simulink model "ModeloNoLineal"  (R2024b)
settings: Solver=VariableStepAuto  StartTime=0.0  StopTime=30  RelTol=1e-3
values from neighbouring files (symbols this model uses):
  B1 = 1200    [ValoresIniciales.m]
  B2 = 500    [ValoresIniciales.m]
  Bt = 10    [ValoresIniciales.m]
  Fs = 0    [ValoresIniciales.m]
  Knl = 1.0e6    (= 1000000)    [ValoresIniciales.m]
  Ks = 16000    [ValoresIniciales.m]    (also in quarter_car_model.m = 48000)
  Kt = 160000    [ValoresIniciales.m]    (also in quarter_car_model.m = 200000)
  Mb = 300    [ValoresIniciales.m]
  Mw = 30    [ValoresIniciales.m]
settings Model: Creator=juanp  LastModifiedBy=juanp

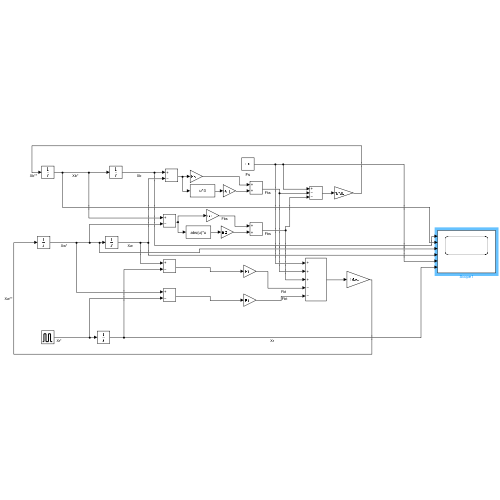
[thumbnail: Simulink's stored preview of the top-level diagram]
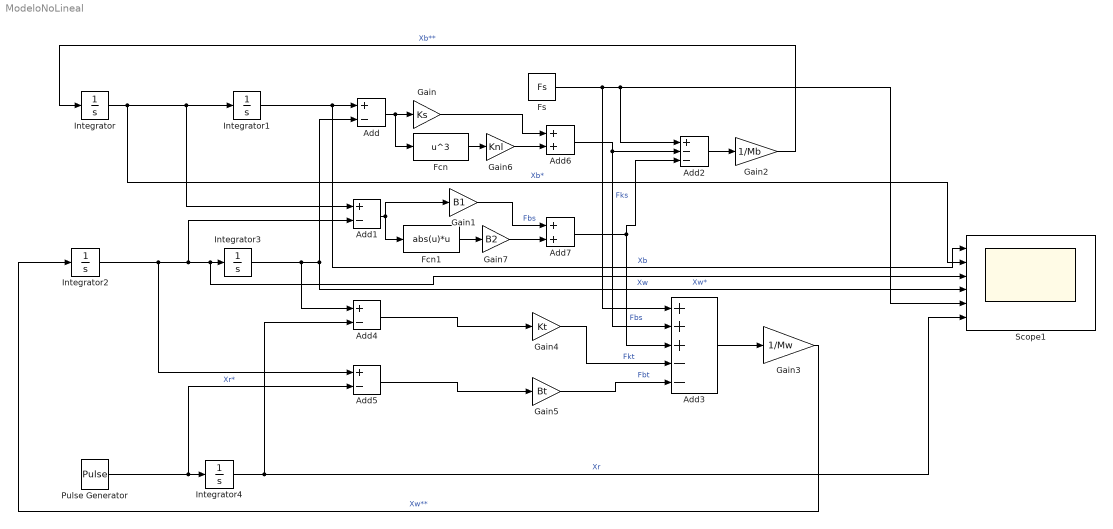
== system ModeloNoLineal ==
  Add{,1,4..5} (4 alike) : Sum  Inputs=+-
  Add2 : Sum  Inputs=+--
  Add3 : Sum  Inputs=+++--
  Add6 : Sum
  Add7 : Sum
  Fcn : Fcn  Expr=u^3
  Fcn1 : Fcn  Expr=abs(u)*u
  Fs : Constant  Value=Fs
  Gain : Gain  Gain=Ks
  Gain1 : Gain  Gain=B1
  Gain2 : Gain  Gain=1/Mb
  Gain3 : Gain  Gain=1/Mw
  Gain4 : Gain  Gain=Kt
  Gain5 : Gain  Gain=Bt
  Gain6 : Gain  Gain=Knl
  Gain7 : Gain  Gain=B2
  Integrator{,1..4} (5 alike) : Integrator
  Pulse Generator : DiscretePulseGenerator  PulseType=Time based  Amplitude=200  Period=10
  Scope1 : Scope  NumInputPorts=6
  wires:
  Fs/1 -> Scope1/5, Add2/1, Add3/1
  Pulse Generator/1 -> Add5/2, Integrator4/1  "Xr*"
  Add1/1 -> Fcn1/1, Gain1/1
  Add2/1 -> Gain2/1
  Add3/1 -> Gain3/1
  Add4/1 -> Gain4/1
  Add7/1 -> Add2/3, Add3/3  "Fbs"
  Gain2/1 -> Integrator/1  "Xb**"
  Add5/1 -> Gain5/1
  Add/1 -> Fcn/1, Gain/1
  Gain4/1 -> Add3/4  "Fkt"
  Integrator3/1 -> Add4/1, Add/2, Scope1/4  "Xw"
  Integrator2/1 -> Scope1/3, Integrator3/1, Add1/2, Add5/1  "Xw*"
  Integrator1/1 -> Scope1/1, Add/1  "Xb"
  Add6/1 -> Add3/2, Add2/2  "Fks"
  Integrator/1 -> Scope1/2, Add1/1, Integrator1/1  "Xb*"
  Gain3/1 -> Integrator2/1  "Xw**"
  Integrator4/1 -> Add4/2, Scope1/6  "Xr"
  Gain5/1 -> Add3/5  "Fbt"
  Gain/1 -> Add6/1
  Gain6/1 -> Add6/2
  Fcn/1 -> Gain6/1
  Gain1/1 -> Add7/1  "Fbs"
  Gain7/1 -> Add7/2
  Fcn1/1 -> Gain7/1
